simulink model "crs_controller"  (R2025b)
settings: Solver=FixedStepDiscrete  StartTime=0.0  StopTime=0.05  FixedStep=Ts  RelTol=1e-3
undefined symbols (not defined in the file): brake_threshold, DiscIntNeverNeededParam, KeyON, Kp, opMode, reqMode, ShiftDrive, target_dec_hold, target_dec_short, target_inc_hold, target_inc_short, throt_max, throt_min, Ts, tsp_max, tsp_min
libraries: simulink x73
(part 2 of 2)

== matlab function crs_controller/DriverSwRequest/decrement/counter/counter ==
  data: in input boolean size=1; out output boolean size=1; CountValue input uint8 size=1
function out = counter(in,CountValue)
%#codegen

persistent cnt;

% initialize
if isempty(cnt)
    cnt = cast(0,'like',CountValue);
end

% if enabled
if in
    % Output true if CountValue is reached
    if cnt >= CountValue
        out = true;
    else
        % Continue counting and output false        
        cnt = cnt + cast(1,'like',CountValue);
        out = false;
    end
else
    % if disabled, output false and reset
    cnt = cast(0,'like',CountValue);
    out = false;
end
